simulink model "realmodel_lqi_newmodel"  (R2019a)
settings: Solver=ode45  StartTime=0.0  StopTime=15  RelTol=1e-3  EnableMultiTasking=on
InitFcn:
  | lin_discr_model_test_new
values from neighbouring files (symbols this model uses):
  C_new = [1 0 0 0; 1 1 0 0]    [lin_discr_model_test_new.m]
  h = 0.01    [lin_discr_model_test_new.m]
  K1_i = K1_lqi(1,5:6)    [lin_discr_model_test_new.m]
  K1_lq = K1_lqi(1,1:4)    [lin_discr_model_test_new.m]
  K2_i = K2_lqi(1,5:6)    [lin_discr_model_test_new.m]
  K2_lq = K2_lqi(1,1:4)    [lin_discr_model_test_new.m]
  K3_i = K3_lqi(1,5:6)    [lin_discr_model_test_new.m]
  K3_lq = K3_lqi(1,1:4)    [lin_discr_model_test_new.m]
  Ts = 0.01    [lin_discr_model_test_new.m]
undefined symbols (not defined in the file or in its folder): A_eq1, A_eq2, A_eq3, A_eq4, adingain, adinoffs, B_eq1, B_eq2, B_eq3, B_eq4, D_eq1, D_eq2, D_eq3, D_eq4, daoutgain, daoutoffs, DiscIntNeverNeededParam, Discrete, K4_i, K4_lq, Time
libraries: ctrlSharedLib x4
settings Model: Creator=rbabuska  LastModifiedBy=jessi
settings DataIOCC: LimitDataPoints=on  SaveFormat=Array  ReturnWorkspaceOutputs=off  SignalLoggingName=sigsOut
settings OptimizationCC: BooleanDataType=off  ExpressionDepthLimit=2147483647  InitFltsAndDblsToZero=on  LifeSpan=inf
settings DebuggingCC: SaveWithParameterizedLinksMsg=none  SignalResolutionControl=TryResolveAllWithWarning  MultiTaskDSMMsg=warning  MultiTaskCondExecSysMsg=none  AllowSymbolicDim=off  StateNameClashWarn=warning  SFUnexpectedBacktrackingDiag=warning  SFNoUnconditionalDefaultTransitionDiag=warning  SFExecutionAtInitializationDiag=none  ArithmeticOperatorsInVariantConditions=warning
settings HardwareCC: ProdBitPerPointer=32  ProdBitPerSizeT=32  ProdBitPerPtrDiffT=32  ProdLargestAtomicFloat=None  ProdIntDivRoundTo=Undefined  ProdEndianess=Unspecified  ProdWordSize=32  ProdHWDeviceType=32-bit Generic  TargetUnknown=on
settings ModelReferenceCC: PropagateSignalLabelsOutOfModel=off
settings SFSimCC: SimUseLocalCustomCode=off
settings RTWCC: RTWUseLocalCustomCode=off
settings CodeAppCC: StateflowObjectComments=on
settings GRTTargetCC: TargetFcnLib=ansi_tfl_tmw.mat  TargetLangStandard=C89/C90 (ANSI)  GeneratePreprocessorConditionals=Disable all  CombineOutputUpdateFcns=off  GRTInterface=on
settings ConfigComp: CovMetricSettings=dw  CovHtmlReporting=on  CovSaveCumulativeToWorkspaceVar=on  CovSaveSingleToWorkspaceVar=on  CovExternalEMLEnable=off

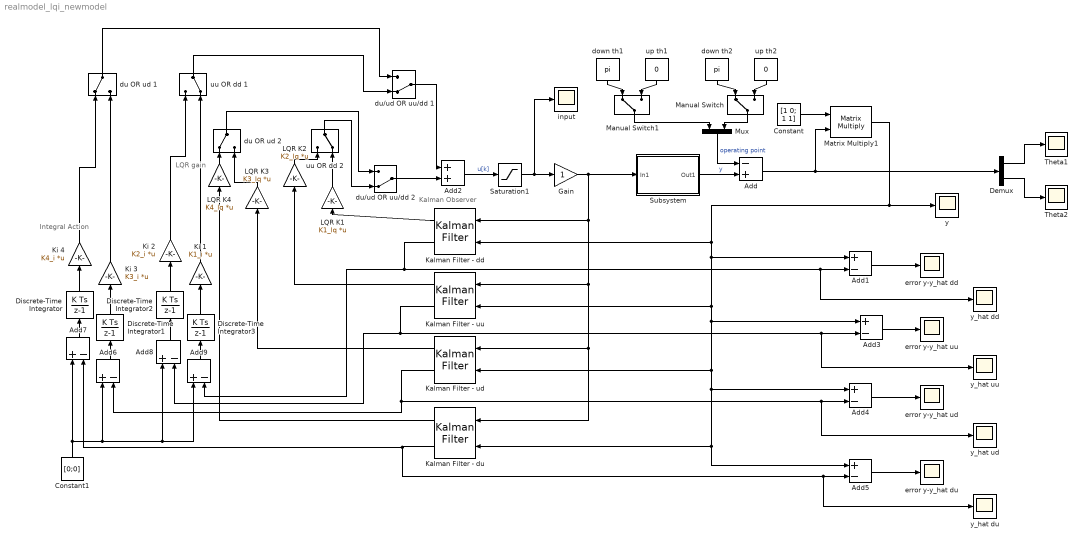
== system realmodel_lqi_newmodel ==
  note: Kalman Observer
  note: LQR gain
  note: Integral Action
  Add : Sum  Inputs=-+
  Add{1,3..9} (8 alike) : Sum  Inputs=+-
  Add2 : Sum
  Constant : Constant  Value=[1 0; 1 1]
  Constant1 : Constant  Value=[0;0]  SampleTime=Ts
  Demux : Demux  Outputs=2
  Discrete-Time Integrator{,1..3} (4 alike) : DiscreteIntegrator  SampleTime=Ts  ICPrevOutput=DiscIntNeverNeededParam  ICPrevScaledInput=DiscIntNeverNeededParam
  Gain : Gain
  Kalman Filter - dd : ctrlSharedLib/Kalman Filter  TimeDomain=Discrete-Time  UseCurrentEstimator=on  ModelSource=Individual A, B, C, D matrices  ModelSourceVariable=sysd1_n  A=A_eq1  B=B_eq1  C=C_new  D=D_eq1  NumberOfStates=1  NumberOfInputs=1  NumberOfOutputs=1  InitialEstimateSource=Dialog  X0=[0;0;0;0]  P0=10  UseK=off  UseGH=off  NumberOfProcessNoiseInputs=1  G=1  TimeInvariantG=on  H=0  TimeInvariantH=on  Q=0.0001*diag([1 1 1 1])  TimeInvariantQ=on  R=0.0001  TimeInvariantR=on  N=0  TimeInvariantN=on  AddInputPort=on  AddEnablePort=off  OutputEstimatedY=on  OutputP=off  Ts=Ts
      settings: SourceProductBaseCode=CT
  Kalman Filter - du : ctrlSharedLib/Kalman Filter  TimeDomain=Discrete-Time  UseCurrentEstimator=on  ModelSource=Individual A, B, C, D matrices  ModelSourceVariable=sysd4_n  A=A_eq4  B=B_eq4  C=C_new  D=D_eq4  NumberOfStates=4  NumberOfInputs=1  NumberOfOutputs=2  InitialEstimateSource=Dialog  X0=[0;0;0;0]  P0=10  UseK=off  UseGH=off  NumberOfProcessNoiseInputs=1  G=1  TimeInvariantG=on  H=0  TimeInvariantH=on  Q=diag([100 100 0.01 0.01])  TimeInvariantQ=on  R=0.0001  TimeInvariantR=on  N=0  TimeInvariantN=on  AddInputPort=on  AddEnablePort=off  OutputEstimatedY=on  OutputP=off  Ts=Ts
      settings: SourceProductBaseCode=CT
  Kalman Filter - ud : ctrlSharedLib/Kalman Filter  TimeDomain=Discrete-Time  UseCurrentEstimator=on  ModelSource=Individual A, B, C, D matrices  ModelSourceVariable=sysd3_n  A=A_eq3  B=B_eq3  C=C_new  D=D_eq3  NumberOfStates=1  NumberOfInputs=1  NumberOfOutputs=1  InitialEstimateSource=Dialog  X0=[0;0;0;0]  P0=10  UseK=off  UseGH=off  NumberOfProcessNoiseInputs=1  G=1  TimeInvariantG=on  H=0  TimeInvariantH=on  Q=diag([100 0.01 10 0.01])  TimeInvariantQ=on  R=0.0001  TimeInvariantR=on  N=0  TimeInvariantN=on  AddInputPort=on  AddEnablePort=off  OutputEstimatedY=on  OutputP=off  Ts=Ts
      settings: SourceProductBaseCode=CT
  Kalman Filter - uu : ctrlSharedLib/Kalman Filter  TimeDomain=Discrete-Time  UseCurrentEstimator=on  ModelSource=Individual A, B, C, D matrices  ModelSourceVariable=sysd2_n  A=A_eq2  B=B_eq2  C=C_new  D=D_eq2  NumberOfStates=1  NumberOfInputs=1  NumberOfOutputs=1  InitialEstimateSource=Dialog  X0=[0;0;0;0]  P0=10  UseK=off  UseGH=off  NumberOfProcessNoiseInputs=1  G=1  TimeInvariantG=on  H=0  TimeInvariantH=on  Q=0.0001*diag([1 1 1 1])  TimeInvariantQ=on  R=0.0001  TimeInvariantR=on  N=0  TimeInvariantN=on  AddInputPort=on  AddEnablePort=off  OutputEstimatedY=on  OutputP=off  Ts=Ts
      settings: SourceProductBaseCode=CT
  Ki 1 : Gain  Gain=K1_i  Multiplication=Matrix(K*u)
  Ki 2 : Gain  Gain=K2_i  Multiplication=Matrix(K*u)
  Ki 3 : Gain  Gain=K3_i  Multiplication=Matrix(K*u)
  Ki 4 : Gain  Gain=K4_i  Multiplication=Matrix(K*u)
  LQR K1 : Gain  Gain=K1_lq  Multiplication=Matrix(K*u)
  LQR K2 : Gain  Gain=K2_lq  Multiplication=Matrix(K*u)
  LQR K3 : Gain  Gain=K3_lq  Multiplication=Matrix(K*u)
  LQR K4 : Gain  Gain=K4_lq  Multiplication=Matrix(K*u)
  Manual Switch : ManualSwitch
  Manual Switch1 : ManualSwitch
  Matrix Multiply1 : Product  Multiplication=Matrix(*)
  Mux : Mux  Inputs=2
  Saturation1 : Saturate  UpperLimit=1  LowerLimit=-1
  Subsystem : Subsystem
      mask Display: disp('Rotational\nPendulum')
  Theta1 : Scope
  Theta2 : Scope
  down th1 : Constant  Value=pi
  down th2 : Constant  Value=pi
  du OR ud 1 : ManualSwitch
  du OR ud 2 : ManualSwitch
  du/ud OR uu/dd 1 : ManualSwitch  CurrentSetting=0
  du/ud OR uu/dd 2 : ManualSwitch  CurrentSetting=0
  error y-y_hat dd : Scope
  error y-y_hat du : Scope
  error y-y_hat ud : Scope
  error y-y_hat uu : Scope
  input : Scope
  up th1 : Constant  Value=0
  up th2 : Constant  Value=0
  uu OR dd 1 : ManualSwitch  CurrentSetting=0
  uu OR dd 2 : ManualSwitch  CurrentSetting=0
  y : Scope
  y_hat dd : Scope
  y_hat du : Scope
  y_hat ud : Scope
  y_hat uu : Scope
  wires:
  Demux/1 -> Theta1/1
  Demux/2 -> Theta2/1
  Add2/1 -> Saturation1/1  "u[k]"
  Subsystem/1(Out1) -> Add/2  "y"
  Add/1 -> Matrix Multiply1/2, Demux/1
  Add1/1 -> error y-y_hat dd/1
  Saturation1/1 -> input/1, Gain/1
  Constant/1 -> Matrix Multiply1/1
  Matrix Multiply1/1 -> Add3/1, Kalman Filter - ud/2, Add4/1, Add5/1, Kalman Filter - du/2, Kalman Filter - uu/2, Add1/1, Kalman Filter - dd/2, y/1
  Mux/1 -> Add/1  "operating point"
  Manual Switch/1 -> Mux/2
  Manual Switch1/1 -> Mux/1
  down th2/1 -> Manual Switch/1
  up th2/1 -> Manual Switch/2
  up th1/1 -> Manual Switch1/2
  down th1/1 -> Manual Switch1/1
  Gain/1 -> Kalman Filter - du/1, Kalman Filter - ud/1, Kalman Filter - uu/1, Kalman Filter - dd/1, Subsystem/1(In1)
  Kalman Filter - dd/1 -> LQR K1/1
  Kalman Filter - uu/1 -> LQR K2/1
  Kalman Filter - ud/1 -> LQR K3/1
  Kalman Filter - du/1 -> LQR K4/1
  LQR K1/1 -> uu OR dd 2/2
  LQR K2/1 -> uu OR dd 2/1
  LQR K4/1 -> du OR ud 2/1
  LQR K3/1 -> du OR ud 2/2
  du/ud OR uu/dd 2/1 -> Add2/2
  du OR ud 2/1 -> du/ud OR uu/dd 2/1
  uu OR dd 2/1 -> du/ud OR uu/dd 2/2
  Kalman Filter - dd/2 -> Add9/2, y_hat dd/1, Add1/2
  Add3/1 -> error y-y_hat uu/1
  Add4/1 -> error y-y_hat ud/1
  Add5/1 -> error y-y_hat du/1
  Kalman Filter - du/2 -> Add7/2, y_hat du/1, Add5/2
  Kalman Filter - ud/2 -> Add6/2, y_hat ud/1, Add4/2
  Kalman Filter - uu/2 -> Add8/2, y_hat uu/1, Add3/2
  Constant1/1 -> Add7/1, Add9/1, Add8/1, Add6/1
  Add7/1 -> Discrete-Time Integrator/1
  du/ud OR uu/dd 1/1 -> Add2/1
  du OR ud 1/1 -> du/ud OR uu/dd 1/1
  uu OR dd 1/1 -> du/ud OR uu/dd 1/2
  Ki 3/1 -> du OR ud 1/2
  Ki 1/1 -> uu OR dd 1/2
  Ki 4/1 -> du OR ud 1/1
  Ki 2/1 -> uu OR dd 1/1
  Discrete-Time Integrator/1 -> Ki 4/1
  Add6/1 -> Discrete-Time Integrator1/1
  Add8/1 -> Discrete-Time Integrator2/1
  Add9/1 -> Discrete-Time Integrator3/1
  Discrete-Time Integrator3/1 -> Ki 1/1
  Discrete-Time Integrator2/1 -> Ki 2/1
  Discrete-Time Integrator1/1 -> Ki 3/1

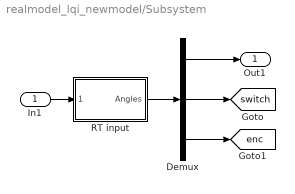
== system realmodel_lqi_newmodel/Subsystem ==
  In1 : Inport
  Demux : Demux  Outputs=[2 4 1]
  RT input : Subsystem  mask{Ts=h, channels=[6 7]}
      mask prompts: Ts "Sample time [s]:"; channels "Channels to read (e.g., [6 7])"
      mask init:
      | hwinit;
      | 
      | % initialize FPGA
      | fugihandle = fugiboard('Open', 'Pendulum1');
      | fugihandle.WatchdogTimeout = 0.5;
      | fugiboard('SetParams', fugihandle);
      | fugiboard('Write', fugihandle, 0, 0, 0, 0);  % dummy write to sync interface board
      | fugiboard('Write', fugihandle, 5, 1, 0, 0);  % reset position, activate relay
      | data = fugiboard('Read', fugihandle);        % get version info from FPGA
      | % model = bitshift(data(1), -5); 
      | % version = bitand(data(1), 31);
      | % disp(sprintf('FPGA setup %d, version %d', model, version)); % for the B&P it should say 1 1, or else there is a problem
      | fugiboard('Write', fugihandle, 0, 1, 0, 0);  % end reset
      | pause(0.1);                         % give relay some time to respond
      mask Display: disp('Rotational\nPendulum')
  Out1 : Outport
  tag scope: enc=global, switch=global
  wires:
  RT input/1(Angles) -> Demux/1
  Demux/1 -> Out1/1
  Demux/2 -> [switch]
  Demux/3 -> [enc]
  In1/1 -> RT input/1(Motors)

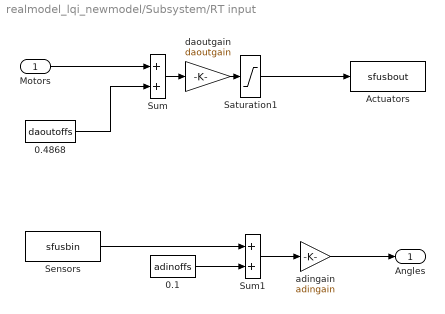
== system realmodel_lqi_newmodel/Subsystem/RT input ==
  Motors : Inport
  0.1 : Constant  Value=adinoffs
  0.4868 : Constant  Value=daoutoffs
  Actuators : S-Function  FunctionName=sfusbout  Parameters=Ts, fugihandle  SFunctionDeploymentMode=off  EnableBusSupport=off
  Saturation1 : Saturate  UpperLimit=10  LowerLimit=-10
  Sensors : S-Function  FunctionName=sfusbin  Parameters=Ts, fugihandle, channels  SFunctionDeploymentMode=off  EnableBusSupport=off
  Sum : Sum  SaturateOnIntegerOverflow=on  InputSameDT=on  OutDataTypeStr=Inherit: Same as first input
  Sum1 : Sum  SaturateOnIntegerOverflow=on  InputSameDT=on  OutDataTypeStr=Inherit: Same as first input
  adingain : Gain  Gain=adingain  SaturateOnIntegerOverflow=on  OutDataTypeStr=Inherit: Same as input  ParamDataTypeStr=Inherit: Same as input
  daoutgain : Gain  Gain=daoutgain  SaturateOnIntegerOverflow=on  OutDataTypeStr=Inherit: Same as input  ParamDataTypeStr=Inherit: Same as input
  Angles : Outport
  wires:
  Sum/1 -> daoutgain/1
  0.4868/1 -> Sum/2
  Motors/1 -> Sum/1
  Sum1/1 -> adingain/1
  0.1/1 -> Sum1/2
  adingain/1 -> Angles/1
  Saturation1/1 -> Actuators/1
  daoutgain/1 -> Saturation1/1
  Sensors/1 -> Sum1/1
